simulink model "Lab4_PID"  (R2022a)
settings: Solver=VariableStepAuto  StartTime=0.0  StopTime=50  RelTol=1e-3
settings Model: Creator=bebawy  LastModifiedBy=bebawy

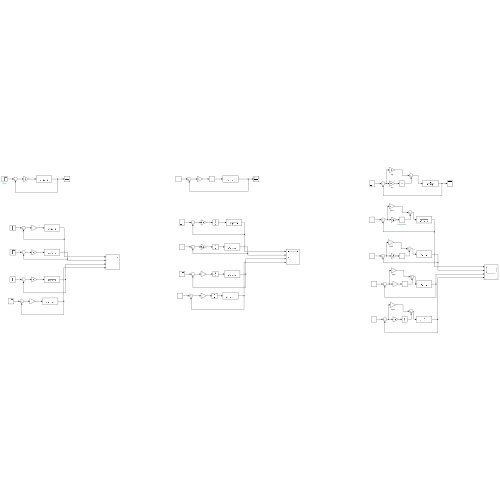
[thumbnail: Simulink's stored preview of the top-level diagram]
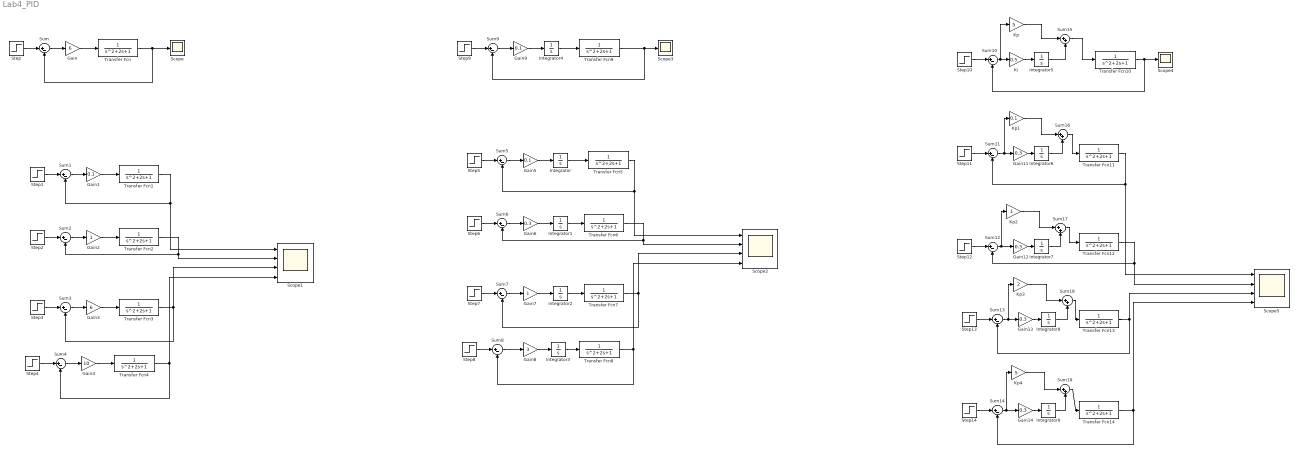
== system Lab4_PID ==
  Gain : Gain  Gain=6
  Gain1 : Gain  Gain=0.1
  Gain{6,11..14} (5 alike) : Gain  Gain=0.3
  Gain2 : Gain
  Gain3 : Gain  Gain=6
  Gain4 : Gain  Gain=10
  Gain5 : Gain  Gain=0.1
  Gain7 : Gain
  Gain8 : Gain  Gain=3
  Gain9 : Gain  Gain=0.1
  Integrator{,1..9} (10 alike) : Integrator
  Ki : Gain  Gain=0.5
  Kp : Gain  Gain=5
  Kp1 : Gain  Gain=0.1
  Kp2 : Gain
  Kp3 : Gain  Gain=2
  Kp4 : Gain  Gain=5
  Scope : Scope
  Scope1 : Scope  NumInputPorts=4
  Scope2 : Scope  NumInputPorts=4
  Scope3 : Scope
  Scope4 : Scope
  Scope5 : Scope  NumInputPorts=4
  Step{,1..14} (15 alike) : Step  SampleTime=0
  Sum{,1..14} (15 alike) : Sum  Inputs=|+-
  Sum{15..19} (5 alike) : Sum  Inputs=|++
  Transfer Fcn{,1..14} (15 alike) : TransferFcn
  wires:
  Sum/1 -> Gain/1
  Gain/1 -> Transfer Fcn/1
  Step/1 -> Sum/1
  Transfer Fcn/1 -> Sum/2, Scope/1
  Transfer Fcn1/1 -> Scope1/1, Sum1/2
  Sum1/1 -> Gain1/1
  Step1/1 -> Sum1/1
  Gain1/1 -> Transfer Fcn1/1
  Step2/1 -> Sum2/1
  Sum2/1 -> Gain2/1
  Gain2/1 -> Transfer Fcn2/1
  Transfer Fcn2/1 -> Scope1/2, Sum2/2
  Sum3/1 -> Gain3/1
  Transfer Fcn3/1 -> Sum3/2, Scope1/3
  Gain3/1 -> Transfer Fcn3/1
  Step3/1 -> Sum3/1
  Sum4/1 -> Gain4/1
  Transfer Fcn4/1 -> Scope1/4, Sum4/2
  Gain4/1 -> Transfer Fcn4/1
  Step4/1 -> Sum4/1
  Transfer Fcn7/1 -> Sum7/2, Scope2/3
  Sum7/1 -> Gain7/1
  Gain7/1 -> Integrator2/1
  Step5/1 -> Sum5/1
  Transfer Fcn5/1 -> Scope2/1, Sum5/2
  Step8/1 -> Sum8/1
  Transfer Fcn8/1 -> Scope2/4, Sum8/2
  Sum8/1 -> Gain8/1
  Step7/1 -> Sum7/1
  Sum6/1 -> Gain6/1
  Gain6/1 -> Integrator1/1
  Gain8/1 -> Integrator3/1
  Transfer Fcn6/1 -> Scope2/2, Sum6/2
  Sum5/1 -> Gain5/1
  Gain5/1 -> Integrator/1
  Step6/1 -> Sum6/1
  Integrator/1 -> Transfer Fcn5/1
  Integrator1/1 -> Transfer Fcn6/1
  Integrator2/1 -> Transfer Fcn7/1
  Integrator3/1 -> Transfer Fcn8/1
  Integrator4/1 -> Transfer Fcn9/1
  Gain9/1 -> Integrator4/1
  Sum9/1 -> Gain9/1
  Step9/1 -> Sum9/1
  Transfer Fcn9/1 -> Scope3/1, Sum9/2
  Step10/1 -> Sum10/1
  Transfer Fcn10/1 -> Scope4/1, Sum10/2
  Ki/1 -> Integrator5/1
  Sum10/1 -> Kp/1, Ki/1
  Step13/1 -> Sum13/1
  Step14/1 -> Sum14/1
  Step11/1 -> Sum11/1
  Gain13/1 -> Integrator8/1
  Transfer Fcn11/1 -> Scope5/1, Sum11/2
  Transfer Fcn13/1 -> Scope5/3, Sum13/2
  Step12/1 -> Sum12/1
  Gain11/1 -> Integrator6/1
  Transfer Fcn12/1 -> Scope5/2, Sum12/2
  Gain14/1 -> Integrator9/1
  Sum11/1 -> Kp1/1, Gain11/1
  Gain12/1 -> Integrator7/1
  Transfer Fcn14/1 -> Scope5/4, Sum14/2
  Integrator5/1 -> Sum15/2
  Sum15/1 -> Transfer Fcn10/1
  Kp/1 -> Sum15/1
  Kp1/1 -> Sum16/1
  Sum16/1 -> Transfer Fcn11/1
  Integrator6/1 -> Sum16/2
  Sum12/1 -> Kp2/1, Gain12/1
  Sum17/1 -> Transfer Fcn12/1
  Integrator7/1 -> Sum17/2
  Kp2/1 -> Sum17/1
  Sum13/1 -> Kp3/1, Gain13/1
  Integrator8/1 -> Sum18/2
  Kp3/1 -> Sum18/1
  Sum18/1 -> Transfer Fcn13/1
  Sum14/1 -> Kp4/1, Gain14/1
  Integrator9/1 -> Sum19/2
  Kp4/1 -> Sum19/1
  Sum19/1 -> Transfer Fcn14/1
